simulink model "my_system"  (R2020a)
settings: Solver=VariableStepAuto  StartTime=0.0  StopTime=10.0  RelTol=1e-3
settings Model: Creator=User  LastModifiedBy=User

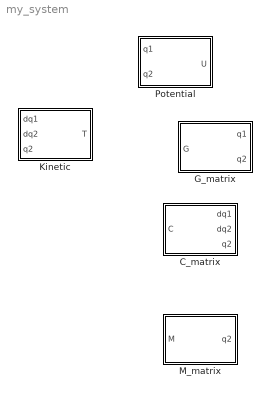
== system my_system ==
  C_matrix : MATLAB Function  TreatAsAtomicUnit=on
  G_matrix : MATLAB Function  TreatAsAtomicUnit=on
  Kinetic : MATLAB Function  TreatAsAtomicUnit=on
  M_matrix : MATLAB Function  TreatAsAtomicUnit=on
  Potential : MATLAB Function  TreatAsAtomicUnit=on

== matlab function my_system/M_matrix ==
  data: q2 input; M output
function M = M_matrix(q2)
%#codegen

%    This function was generated by the Symbolic Math Toolbox version 8.5.
%    04-Nov-2022 18:56:12

t2 = cos(q2);
t3 = t2./2.0;
t4 = t3+3.341666666666667e-1;
M = reshape([t2+1.668333333333333,t4,t4,3.341666666666667e-1],[2,2]);

== matlab function my_system/G_matrix ==
  data: q1 input; G output; q2 input
function G = G_matrix(q1,q2)
%#codegen

%    This function was generated by the Symbolic Math Toolbox version 8.5.
%    04-Nov-2022 18:56:13

t2 = q1+q2;
t3 = cos(t2);
t4 = t3.*(9.81e+2./2.0e+2);
G = [t4+cos(q1).*1.4715e+1;t4];

== matlab function my_system/Kinetic ==
  data: dq1 input; T output; dq2 input; q2 input
function T = Kinetic(dq1,dq2,q2)
%#codegen

%    This function was generated by the Symbolic Math Toolbox version 8.5.
%    04-Nov-2022 18:56:13

t2 = cos(q2);
t3 = t2./2.0;
t4 = t3+3.341666666666667e-1;
T = dq2.*(dq2.*1.670833333333333e-1+(dq1.*t4)./2.0)+dq1.*((dq2.*t4)./2.0+(dq1.*(t2+1.668333333333333))./2.0);

== matlab function my_system/Potential ==
  data: q1 input; U output; q2 input
function U = Potential(q1,q2)
%#codegen

%    This function was generated by the Symbolic Math Toolbox version 8.5.
%    04-Nov-2022 18:56:13

U = sin(q1+q2).*(9.81e+2./2.0e+2)+sin(q1).*1.4715e+1;

== matlab function my_system/C_matrix ==
  data: dq1 input; C output; dq2 input; q2 input
function C = C_matrix(dq1,dq2,q2)
%#codegen

%    This function was generated by the Symbolic Math Toolbox version 8.5.
%    04-Nov-2022 18:56:12

t2 = sin(q2);
t3 = (dq1.*t2)./2.0;
t4 = (dq2.*t2)./2.0;
t5 = -t4;
C = reshape([t5,t3,-t3+t5,0.0],[2,2]);
